simulink model "PID_quad"  (Simulink 8.1)
settings: Solver=ode45  StartTime=0.0  StopTime=10.0  RelTol=1e-10
values from neighbouring files (symbols this model uses):
  bm = 5106.8    [quad_init.m]
  d = 0.16    [quad_init.m]
  g = 9.8    [quad_init.m]
  km = 342.4    [quad_init.m]
  m = 0.835    [quad_init.m]
undefined symbols (not defined in the file or in its folder): K_pitch, K_roll, K_yaw, Td_pitch, Td_roll, Td_yaw, Ti_pitch, Ti_roll, Ti_yaw
libraries: dspinverses x1, quad_lib x1
settings Model: Creator=diogo  LastModifiedBy=diogo
settings DebuggingCC: StrictBusMsg=Warning

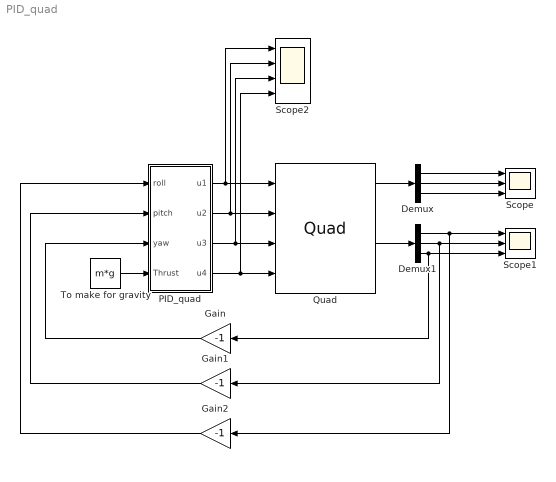
== system PID_quad ==
  Demux : Demux  Outputs=3
  Demux1 : Demux  Outputs=3
  Gain : Gain  Gain=-1
  Gain1 : Gain  Gain=-1
  Gain2 : Gain  Gain=-1
  PID_quad : Subsystem
  Quad : quad_lib/Quad
  Scope : Scope  NumInputPorts=3
      settings: YMin=-5~-5~-5  YMax=5~5~5
  Scope1 : Scope  NumInputPorts=3
      settings: TimeRange=100  YMin=-4~-2~-4  YMax=4~2~4
  Scope2 : Scope  NumInputPorts=4
      settings: TimeRange=10  YMin=-10000000000000~-10000000000000~-5000000000000~-5000000000000  YMax=5000000000000~5000000000000~10000000000000~10000000000000  SaveName=ScopeData2
  To make for gravity : Constant  Value=m*g
  wires:
  PID_quad/1(" u1") -> Scope2/1, Quad/1
  PID_quad/2(" u2") -> Scope2/2, Quad/2
  PID_quad/3(" u3") -> Scope2/3, Quad/3
  PID_quad/4(" u4") -> Scope2/4, Quad/4
  Gain/1 -> PID_quad/3(yaw)
  Gain1/1 -> PID_quad/2(pitch)
  Gain2/1 -> PID_quad/1(roll)
  To make for gravity/1 -> PID_quad/4(Thrust)
  Quad/1 -> Demux/1
  Quad/3 -> Demux1/1
  Demux/1 -> Scope/1
  Demux/2 -> Scope/2
  Demux/3 -> Scope/3
  Demux1/1 -> Gain2/1, Scope1/1
  Demux1/2 -> Gain1/1, Scope1/2
  Demux1/3 -> Gain/1, Scope1/3

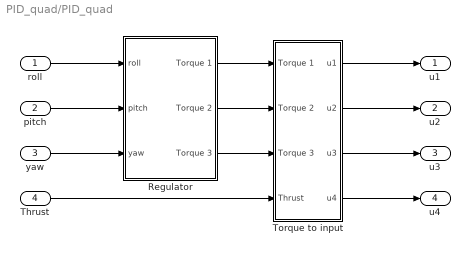
== system PID_quad/PID_quad ==
  roll : Inport
  pitch : Inport  Port=2
  yaw : Inport  Port=3
  Thrust : Inport  Port=4
  Regulator : Subsystem
  Torque to input : Subsystem
  " u1" : Outport
  " u2" : Outport  Port=2
  " u3" : Outport  Port=3
  " u4" : Outport  Port=4
  wires:
  roll/1 -> Regulator/1(roll)
  pitch/1 -> Regulator/2(pitch)
  yaw/1 -> Regulator/3(yaw)
  Torque to input/1(" u1") -> " u1"/1
  Torque to input/2(" u2") -> " u2"/1
  Torque to input/3(" u3") -> " u3"/1
  Torque to input/4(" u4") -> " u4"/1
  Regulator/1(" Torque 1") -> Torque to input/1(Torque 1)
  Regulator/2(" Torque 2") -> Torque to input/2(Torque 2)
  Regulator/3(" Torque 3") -> Torque to input/3(Torque 3)
  Thrust/1 -> Torque to input/4(Thrust)

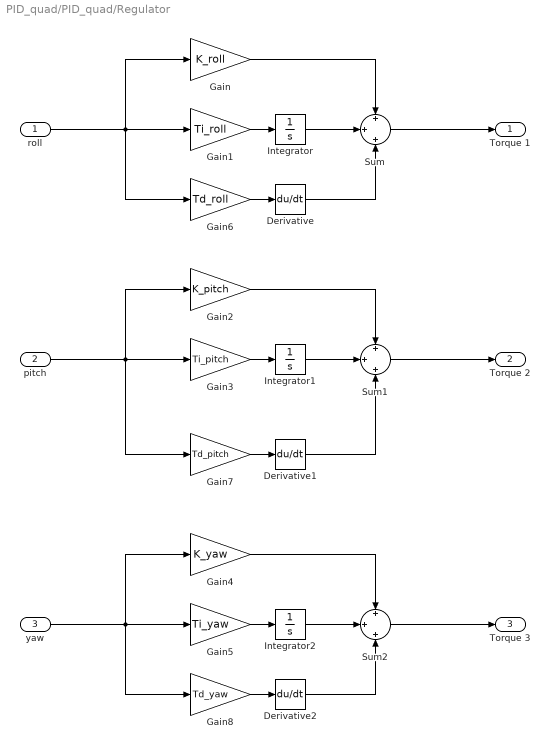
== system PID_quad/PID_quad/Regulator ==
  roll : Inport
  pitch : Inport  Port=2
  yaw : Inport  Port=3
  Derivative : Derivative
  Derivative1 : Derivative
  Derivative2 : Derivative
  Gain : Gain  Gain=K_roll
  Gain1 : Gain  Gain=Ti_roll
  Gain2 : Gain  Gain=K_pitch
  Gain3 : Gain  Gain=Ti_pitch
  Gain4 : Gain  Gain=K_yaw
  Gain5 : Gain  Gain=Ti_yaw
  Gain6 : Gain  Gain=Td_roll
  Gain7 : Gain  Gain=Td_pitch
  Gain8 : Gain  Gain=Td_yaw
  Integrator : Integrator
  Integrator1 : Integrator
  Integrator2 : Integrator
  Sum : Sum  Inputs=+|+|+
  Sum1 : Sum  Inputs=+|+|+
  Sum2 : Sum  Inputs=+|+|+
  " Torque 1" : Outport
  " Torque 2" : Outport  Port=2
  " Torque 3" : Outport  Port=3
  wires:
  roll/1 -> Gain1/1, Gain/1, Gain6/1
  Gain/1 -> Sum/1
  Gain1/1 -> Integrator/1
  Integrator/1 -> Sum/2
  Sum/1 -> " Torque 1"/1
  pitch/1 -> Gain3/1, Gain2/1, Gain7/1
  Gain2/1 -> Sum1/1
  Gain3/1 -> Integrator1/1
  Integrator1/1 -> Sum1/2
  yaw/1 -> Gain5/1, Gain4/1, Gain8/1
  Gain4/1 -> Sum2/1
  Gain5/1 -> Integrator2/1
  Integrator2/1 -> Sum2/2
  Sum1/1 -> " Torque 2"/1
  Sum2/1 -> " Torque 3"/1
  Gain6/1 -> Derivative/1
  Derivative/1 -> Sum/3
  Gain7/1 -> Derivative1/1
  Derivative1/1 -> Sum1/3
  Gain8/1 -> Derivative2/1
  Derivative2/1 -> Sum2/3

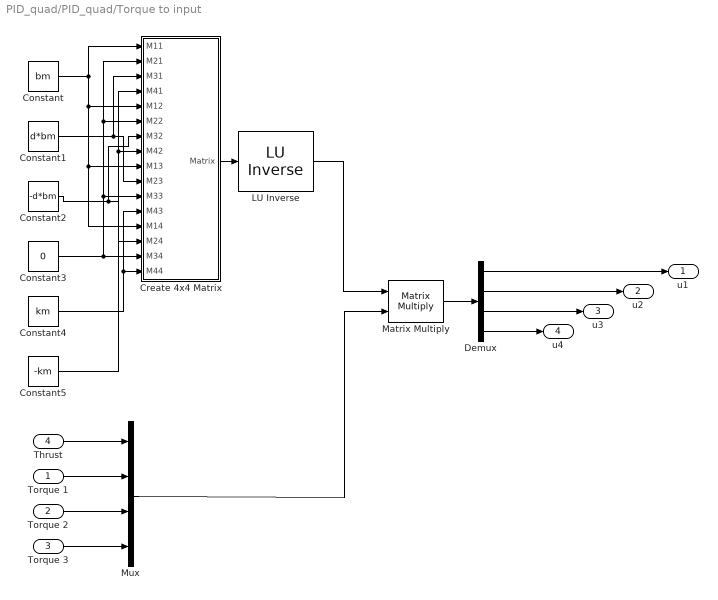
== system PID_quad/PID_quad/Torque to input ==
  Torque 1 : Inport
  Torque 2 : Inport  Port=2
  Torque 3 : Inport  Port=3
  Thrust : Inport  Port=4
  " LU Inverse" : dspinverses/ LU Inverse
  Constant : Constant  Value=bm
  Constant1 : Constant  Value=d*bm
  Constant2 : Constant  Value=-d*bm
  Constant3 : Constant  Value=0
  Constant4 : Constant  Value=km
  Constant5 : Constant  Value=-km
  Create 4x4 Matrix : Subsystem  AncestorBlock=aerolibutil/Create 3x3 Matrix  mask(Create 3x3 Matrix){}
      mask help:
      | Create a 3-by-3 matrix from nine input values. Each input corresponds to an element of the matrix.
      |
      | For example, the input labeled A21 is the entry in the second row and first column of the matrix.
      mask init:
      | aeroicon('aeroblk');
      mask Help: eval('asbhelp(''create_threebythree_matrix'')');
  Demux : Demux
  Matrix Multiply : Product  Multiplication=Matrix(*)
  Mux : Mux
  " u1" : Outport
  " u2" : Outport  Port=2
  " u3" : Outport  Port=3
  " u4" : Outport  Port=4
  wires:
  Thrust/1 -> Mux/1
  Torque 1/1 -> Mux/2
  Torque 2/1 -> Mux/3
  Torque 3/1 -> Mux/4
  Constant/1 -> Create 4x4 Matrix/1(M11), Create 4x4 Matrix/5(M12), Create 4x4 Matrix/9(M13), Create 4x4 Matrix/13(M14)
  Constant3/1 -> Create 4x4 Matrix/2(M21), Create 4x4 Matrix/6(M22), Create 4x4 Matrix/11(M33), Create 4x4 Matrix/15(M34)
  Constant1/1 -> Create 4x4 Matrix/10(M23), Create 4x4 Matrix/3(M31)
  Constant2/1 -> Create 4x4 Matrix/14(M24), Create 4x4 Matrix/7(M32)
  Constant4/1 -> Create 4x4 Matrix/12(M43), Create 4x4 Matrix/16(M44)
  Constant5/1 -> Create 4x4 Matrix/4(M41), Create 4x4 Matrix/8(M42)
  Create 4x4 Matrix/1(Matrix) -> " LU Inverse"/1
  " LU Inverse"/1 -> Matrix Multiply/1
  Mux/1 -> Matrix Multiply/2
  Matrix Multiply/1 -> Demux/1
  Demux/1 -> " u1"/1
  Demux/2 -> " u2"/1
  Demux/3 -> " u3"/1
  Demux/4 -> " u4"/1

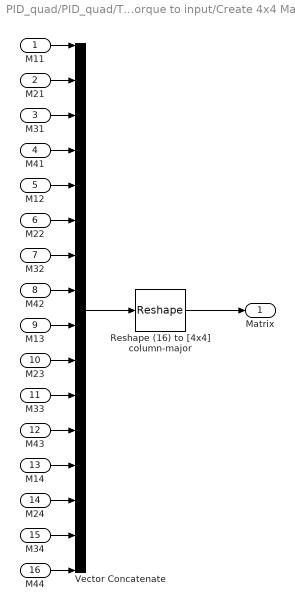
== system PID_quad/PID_quad/Torque to input/Create 4x4 Matrix ==
  M11 : Inport  PortDimensions=1
  M21 : Inport  Port=2  PortDimensions=1
  M31 : Inport  Port=3  PortDimensions=1
  M41 : Inport  Port=4  PortDimensions=1
  M12 : Inport  Port=5  PortDimensions=1
  M22 : Inport  Port=6  PortDimensions=1
  M32 : Inport  Port=7  PortDimensions=1
  M42 : Inport  Port=8  PortDimensions=1
  M13 : Inport  Port=9  PortDimensions=1
  M23 : Inport  Port=10  PortDimensions=1
  M33 : Inport  Port=11  PortDimensions=1
  M43 : Inport  Port=12  PortDimensions=1
  M14 : Inport  Port=13  PortDimensions=1
  M24 : Inport  Port=14  PortDimensions=1
  M34 : Inport  Port=15  PortDimensions=1
  M44 : Inport  Port=16  PortDimensions=1
  Reshape (16) to [4x4] column-major : Reshape  OutputDimensionality=Customize  OutputDimensions=[4,4]
  Vector Concatenate : Concatenate  NumInputs=16
  Matrix : Outport  PortDimensions=[4 4]
  wires:
  Vector Concatenate/1 -> Reshape (16) to [4x4] column-major/1
  M11/1 -> Vector Concatenate/1
  M21/1 -> Vector Concatenate/2
  M31/1 -> Vector Concatenate/3
  M41/1 -> Vector Concatenate/4
  M12/1 -> Vector Concatenate/5
  Reshape (16) to [4x4] column-major/1 -> Matrix/1
  M13/1 -> Vector Concatenate/9
  M22/1 -> Vector Concatenate/6
  M32/1 -> Vector Concatenate/7
  M23/1 -> Vector Concatenate/10
  M33/1 -> Vector Concatenate/11
  M42/1 -> Vector Concatenate/8
  M43/1 -> Vector Concatenate/12
  M14/1 -> Vector Concatenate/13
  M24/1 -> Vector Concatenate/14
  M34/1 -> Vector Concatenate/15
  M44/1 -> Vector Concatenate/16
